simulink model "projects5"  (R2022b)
settings: Solver=FixedStepAuto  StartTime=0.0  StopTime=100.0  RelTol=1e-3  EnableMultiTasking=on
libraries: raspberrypiAVlib x5, audiosources x2
settings Model: ExplicitPartitioning=on  Creator=tatan  LastModifiedBy=tatan
settings SolverCC: AllowMultiTaskInputOutput=on  ConcurrentTasks=on  PositivePriorityOrder=on  AutoInsertRateTranBlk=on
settings OptimizationCC: EnhancedBackFolding=on  PassReuseOutputArgsAs=Individual arguments  ZeroExternalMemoryAtStartup=off  ZeroInternalMemoryAtStartup=off  MaxStackSize=100000  OptimizeBlockOrder=speed  DifferentSizesBufferReuse=on  OptimizationCustomize=off  EfficientTunableParamExpr=on
settings DebuggingCC: ParameterTunabilityLossMsg=error
settings HardwareCC: ProdBitPerPointer=32  ProdBitPerSizeT=32  ProdBitPerPtrDiffT=32  ProdLargestAtomicInteger=Long  ProdLargestAtomicFloat=Double  ProdWordSize=32  ProdLongLongMode=on  ProdHWDeviceType=ARM Compatible->ARM Cortex  UseEmbeddedCoderFeatures=off
settings RTWCC: Description=Embedded Coder  SystemTargetFile=ert.tlc  HardwareBoard=Raspberry Pi  TLCOptions="-aInlineSetEventsForThisBaseRateFcn=TLC_FALSE -aSuppressMultiTaskScheduler=TLC_FALSE  -aRateBasedStepFcn=0"  TemplateMakefile=ert_default_tmf  Toolchain=GNU GCC Embedded Linux  BuildConfiguration=Faster Runs
settings CodeAppCC: ForceParamTrailComments=on  IgnoreCustomStorageClasses=off  OperatorAnnotations=on  SimulinkDataObjDesc=on  SFDataObjDesc=on  InsertBlockDesc=on
settings ERTTargetCC: SupportNonInlinedSFcns=on  SupportVariableSizeSignals=on  ExtModeTransport=2  ExtModeStaticAlloc=on  ExtModeMexFile=ext_xcp  ExtModeIntrfLevel=Level2 - Open

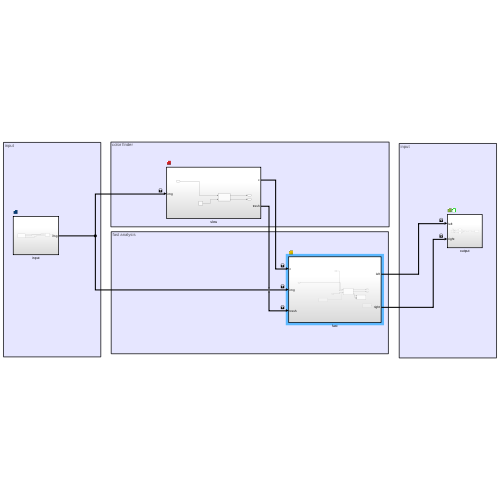
[thumbnail: Simulink's stored preview of the top-level diagram]
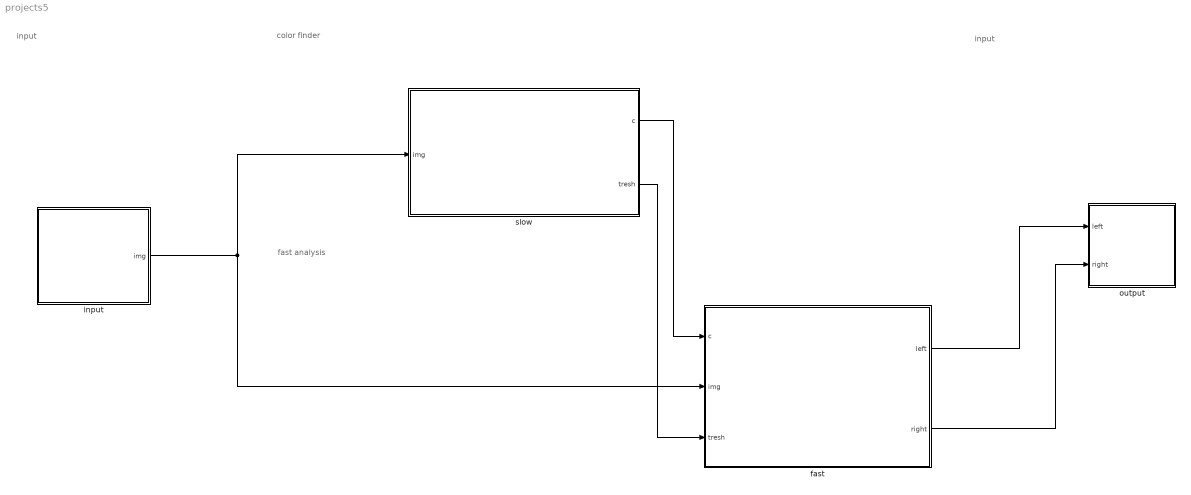
== system projects5 ==
  note: input
  note: color finder
  note: fast analysis
  note: input
  fast : Subsystem  TreatAsAtomicUnit=on
  input : Subsystem  TreatAsAtomicUnit=on
  output : Subsystem  TreatAsAtomicUnit=on
  slow : Subsystem  TreatAsAtomicUnit=on
  wires:
  slow/1(c) -> fast/1(c)
  input/1(img) -> fast/2(img), slow/1(img)
  slow/2(tresh) -> fast/3(tresh)
  fast/1(left) -> output/1(left)
  fast/2(right) -> output/2(right)

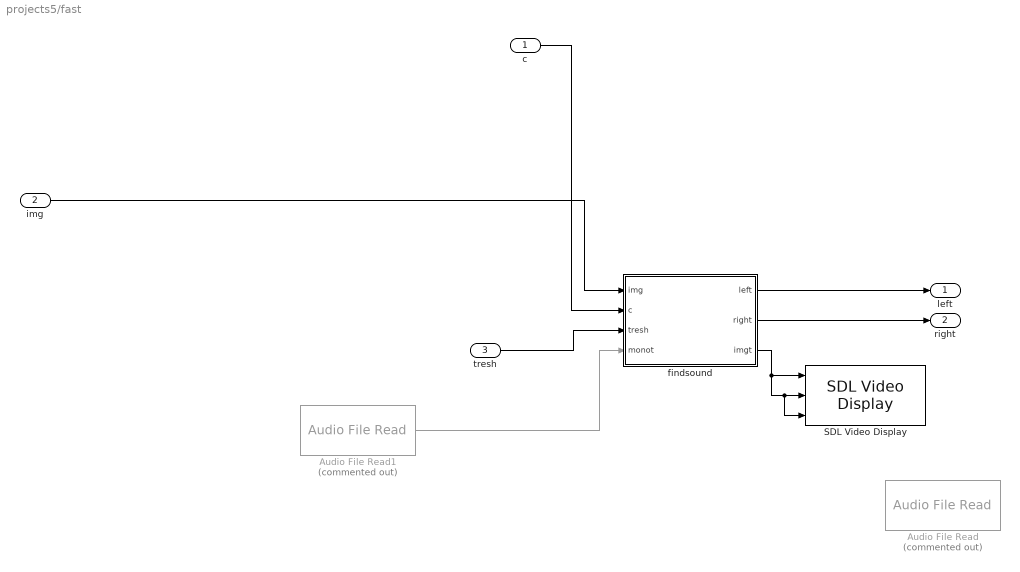
== system projects5/fast ==
  c : Inport
  img : Inport  Port=2
  tresh : Inport  Port=3
  Audio File Read : raspberrypiAVlib/Audio File Read  Commented=on  FileName=helicopter.wav  PlayCount=Inf  OutputEOFIndicator=off  SamplesPerFrame=4410
  Audio File Read1 : raspberrypiAVlib/Audio File Read  Commented=on  FileName=/home/tatan/DossierSyncro/EURECOM/projet/multicoreproject/Hold-the-Line.wav  PlayCount=Inf  OutputEOFIndicator=off  SamplesPerFrame=4410
  SDL Video Display : raspberrypiAVlib/SDL Video Display  title=SDL Video Display  pixelFormat=RGB  pixelOrder=Planar  rowMajor=on  blockPlatform=Raspberry Pi
  findsound : MATLAB Function  TreatAsAtomicUnit=on
  left : Outport
  right : Outport  Port=2
  wires:
  img/1 -> findsound/1(img)
  c/1 -> findsound/2(c)
  tresh/1 -> findsound/3(tresh)
  findsound/3(imgt) -> SDL Video Display/3, SDL Video Display/2, SDL Video Display/1
  Audio File Read1/1 -> findsound/4(monot)
  findsound/2(right) -> right/1
  findsound/1(left) -> left/1

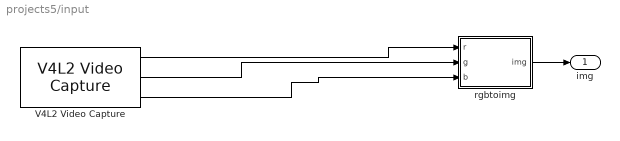
== system projects5/input ==
  V4L2 Video Capture : raspberrypiAVlib/V4L2 Video Capture  DeviceName=/dev/video0  Resolution=320x240  CustomResolution=[ 320, 240 ]  PixelFormat=RGB  SampleTime=0.1  pixelOrder=planar  simOutput=Colorbars  imSizeSelection=320x240  imSize=[640, 480]  roi=[0, 0, 640, 480]  m_devName='/dev/video0'  blockPlatform=LINUX  HorizontalFlip=off  VerticalFlip=off  Brightness=0.5  Saturation=0.5  Contrast=0.5  Sharpness=0.5  CameraPan=0  CameraTilt=0  CameraZoom=0.5  EnableManualFocus=on  ManualFocus=0.5
  rgbtoimg : MATLAB Function  TreatAsAtomicUnit=on
  img : Outport
  wires:
  rgbtoimg/1(img) -> img/1
  V4L2 Video Capture/2 -> rgbtoimg/2(g)
  V4L2 Video Capture/1 -> rgbtoimg/1(r)
  V4L2 Video Capture/3 -> rgbtoimg/3(b)

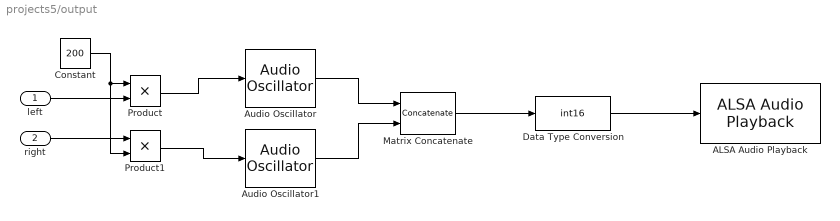
== system projects5/output ==
  left : Inport
  right : Inport  Port=2
  ALSA Audio Playback : raspberrypiAVlib/ALSA Audio Playback  deviceStr='plughw:1,0'  sampleRateEnum=44100  queueDuration=0.5  blockPlatform=LINUX
  Audio Oscillator : audiosources/Audio Oscillator  FrequencyPort=off  Frequency=100  AmplitudePort=on  Amplitude=1  DCOffsetPort=off  PhaseOffset=0  DCOffset=0  WidthPort=off  Width=1  DutyCyclePort=off  DutyCycle=0.5  SampsPerFrame=2048  Fs=44100  OutputDataType=double  SimulateUsing=Code generation
      settings: SignalType=square
  Audio Oscillator1 : audiosources/Audio Oscillator  FrequencyPort=off  Frequency=100  AmplitudePort=on  Amplitude=1  DCOffsetPort=off  PhaseOffset=0  DCOffset=0  WidthPort=off  Width=1  DutyCyclePort=off  DutyCycle=0.5  SampsPerFrame=2048  Fs=44100  OutputDataType=double  SimulateUsing=Code generation
      settings: SignalType=square
  Constant : Constant  Value=200
  Data Type Conversion : DataTypeConversion  OutDataTypeStr=int16  SaturateOnIntegerOverflow=off  RndMeth=Floor
  Matrix Concatenate : Concatenate  Mode=Multidimensional array  ConcatenateDimension=2
  Product : Product
  Product1 : Product
  wires:
  Audio Oscillator/1 -> Matrix Concatenate/1
  Audio Oscillator1/1 -> Matrix Concatenate/2
  Matrix Concatenate/1 -> Data Type Conversion/1
  Data Type Conversion/1 -> ALSA Audio Playback/1
  right/1 -> Product1/1
  left/1 -> Product/2
  Constant/1 -> Product1/2, Product/1
  Product/1 -> Audio Oscillator/1
  Product1/1 -> Audio Oscillator1/1

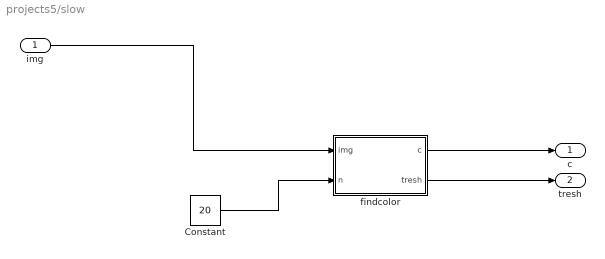
== system projects5/slow ==
  img : Inport
  Constant : Constant  Value=20
  findcolor : MATLAB Function  TreatAsAtomicUnit=on
  c : Outport
  tresh : Outport  Port=2
  wires:
  Constant/1 -> findcolor/2(n)
  findcolor/1(c) -> c/1
  img/1 -> findcolor/1(img)
  findcolor/2(tresh) -> tresh/1

== matlab function projects5/input/rgbtoimg ==
  data: r input; img output; g input; b input
function img= rgbtoimg(r,g,b)
    S = size(r);
    %As in matlab we deal with images with dimentions (n,m,3), and that
    %simulink input is 3 (n,m) image, we transpose the input to match with
    %the matlab code
    imgt=zeros(S(1,1),S(1,2),3);
    imgt(:,:,1) = r(:,:);
    imgt(:,:,2) = g(:,:);
    imgt(:,:,3) = b(:,:);

    %We apply some average filter to make the k mean easier
    h = fspecial("average",[18,18]);
    imgt(:,:,1) = imfilter(imgt(:,:,1),h);
    imgt(:,:,2) = imfilter(imgt(:,:,2),h);
    imgt(:,:,3) = imfilter(imgt(:,:,3),h);
img = uint8(imgt);

== matlab function projects5/slow/findcolor ==
  data: img input; c output; n input; tresh output
function [c,tresh] = findcolor(img,n)
    [img,map,D] = quantize(img,n); %quantizing the image

    % Calculate every fit error for each linear regression 
    index = 0;
    listlen = [];
    listerr = [];

    for i=1:n
        [therror,len] = regressionlineair(img,i);
        listerr = [listerr therror];
        listlen = [listlen len];
    end
    minerror = max(listerr, [], 'all');
    for i=1:n
        if listerr(1,i)<minerror & listlen(1,i)~=max(listlen,[],'all') 
            index = i;
            linelen = listlen(1,i);
            minerror = listerr(1,i)/(log(linelen));
        end
    end

    
    %Here we have the right index
    index;
    D(:,index);
    ct = map(index,:);
    c = ct;
    S = size(img);
    min = -1;
    %And then you choose the biggest sphere possible that contain the only 
    %color specified by index
    for i=1:n
        if i~=index  
            for x=1:S(1,1)
                    for y=1:S(1,2)
                        if img(x,y)==i
                            if min ~= -1
                                if sqrt(D(x*y, i))<min
                                    min = sqrt(D(x*y, i));
                                end
                            end
                            min = sqrt(D(x*y, i));
                        end
                    end
            end
        end
    end
    tresh = min;
end

function [coef,len] = regressionlineair(img, i)
    S = size(img);
    Points = [];
    for l=1:S(1,1)
       Points = [ Points trouvermilieux(img,l,i)];
    end
    x = Points(1,:);
    x = transpose(x);
    s = size(x);
    un = ones(s(1,1),1);
    y = Points(2,:);
    y = transpose(y);
    x = double(x);
    y = double(y);
    [p,S] = polyfit(x,y,1);
    f = polyval(p,x);
    SP = size(Points);
    %calculate the fit error ponderate by the square of the line length
    b = sum((y-f).^2);
    %b% = sum((y-f).^2)/SP(1,2);
    %b = sum((y-f).^2)*log(SP(1,2));
    coef = b;
    len = SP(1,2);
end


function pix = trouvermilieux(img, l, i)
    %for each same colors segment of ligne i, find a middle point
    S = size(img);
    c = 1;
    temp = [];
    while c<S(1,2)
        while img(l,c)~=i & c < S(1,2)
            c=c+1;
        end

        debut = c;
        while img(l,c)==i & c < S(1,2)
            c=c+1;
        end
        fin = int16(c-1);
        if img(l,debut)==i & img(l,fin)==i
            vec = [l int16((debut+fin)/2)];
            vec = transpose(vec);
            temp = [ temp vec];
        end
    end
    pix = temp;
end

%% This is the code that give a proof that the matlab uint8() function is a random function. 
% function [img,map,D] = quantize(rgb,k)
% S=size(rgb);
% tmp = ones(3,S(1,1)*S(1,2));
% for l=1:S(1,1)
%     tmp(:,(l-1)*S(1,2)+1:l*S(1,2))=transpose(squeeze(rgb(l,:,:)));
% end
% [idx,C,sumd,D] = kmeans(transpose(tmp),k);
% idx;
% C;
% sumd;
% imgt = ones(S(1,1),S(1,2));
% 
% for i=1:S(1,1)*S(1,2)
%     imgt(uint32(i/S(1,2))+1,mod(i,S(1,2))+1) = idx(i);
% end
% size(imgt);
% %mapt = int32(C);
% imgt;
% imgt(S(1,1)+1,:) = [];
% %imgt = medfilt2(imgt,[8,8]);
% 
% img = uint8(imgt);
% map = uint8(C);
% end
% 

function [img,map,D] = quantize(rgb,k)
S=size(rgb);
tmp = ones(3,S(1,1)*S(1,2));
%get the list of all pixels of the image
for l=1:S(1,1)
    tmp(:,(l-1)*S(1,2)+1:l*S(1,2))=transpose(squeeze(rgb(l,:,:)));
end
[idx,C,~,D] = kmeans(transpose(tmp),k); % compute a k mean function
imgt = ones(S(1,1),S(1,2));

for i=1:(S(1,1)-1)*S(1,2)
    imgt(uint32(i/S(1,2))+1,mod(i,S(1,2))+1) = idx(i);
end
size(imgt);
size(rgb);
img = imgt;
%map = uint8(C);%mieux vaut garder la precision
map = C;
end

== matlab function projects5/fast/findsound ==
  data: img input; left output; right output; c input; tresh input; imgt output; monot input

function [left, right, imgt] = findsound(img,c,tresh, monot)
%delete all the non line color imager and put the line in full white
S = size(img);
for l=1:S(1,1)
    for x=1:S(1,2)
        tp=img(l,x,:);
        if manorm(double([tp(1),tp(2),tp(3)])-c(1,:))>tresh
            img(l,x,:) = [0,0,0];
        else
            img(l,x,:) = [255,255,255];
        end

    end
end

%grayify the image and process simple median filter to make sampling more
%precise
img = rgb2gray(uint8(img));
img = medfilt2(img,[16,16]);

imgt = img;
%calculate the line angle with the vertical
coef=regressionlineair(img);
angle = ( atan(abs(coef))+pi/2)*sign(coef);
angle * 180/pi;
%output amplitudes ratios for left and right based on trigonometriques
%proportions in order that the sum made 1
if angle > pi/4
   left = 0;
   right = 1;
elseif angle < -pi/4
   left = 1;
   right = 0;
else
   left = sin((angle+pi/4))^2;
   right = cos(angle+pi/4)^2;
end
end



function coef = regressionlineair(img)
    %do some linear regression and return the line angle
    S = size(img);
    Points = [];
    for l=1:S(1,1)
       Points = [ Points trouvermilieux(img,l)];
    end
    x = Points(1,:);
    x = transpose(x);
    s = size(x);
    un = ones(s(1,1),1);
    y = Points(2,:);
    y = transpose(y);
    x = double(x);
    y = double(y);
    p = polyfit(x,y,1);
    coef = p(1,1);
end


function pix = trouvermilieux(img, l)
    %find all middles in same colored segments
    S = size(img);
    c = 1;
    temp = [];
    while c<S(1,2)
        while img(l,c,:)==0 & c < S(1,2)
            c=c+1;
        end

        debut = c;
        while img(l,c,:)>0 & c < S(1,2)
            c=c+1;
        end
        fin = int32(c-1);
        if c < S(1,2)
            vec = [l int32((debut+fin)/2)];
            vec = transpose(vec);
            temp = [ temp vec];
        end
        
    end
    pix = temp;
end

function v = manorm(u)
    %basic eucledian norm
    v = sqrt(double(u(1,1).^2+u(1,2).^2+u(1,3).^2));
end
